simulink model "LeaderFollower"  (R2016a)
settings: Solver=VariableStepAuto  StartTime=0.0  StopTime=inf  RelTol=1e-3
settings Model: Creator=ece446  LastModifiedBy=ece446

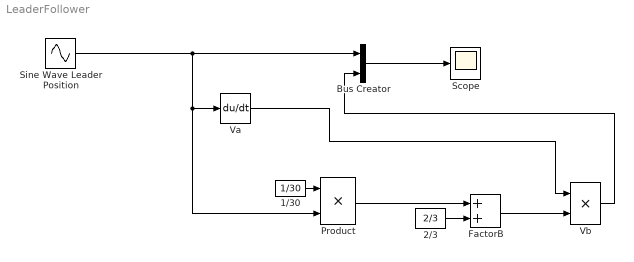
== system LeaderFollower ==
  1/30 : Constant  Value=1/30
  2/3 : Constant  Value=2/3
  Bus Creator : BusCreator  Inputs=2
  FactorB : Sum
  Product : Product
  "Scope " : Scope
  Sine Wave Leader Position : Sin  SampleTime=0
  Va : Derivative  CoefficientInTFapproximation=0
  Vb : Product
  wires:
  Sine Wave Leader Position/1 -> Bus Creator/1, Product/2, Va/1
  Va/1 -> Vb/1
  1/30/1 -> Product/1
  Product/1 -> FactorB/1
  2/3/1 -> FactorB/2
  FactorB/1 -> Vb/2
  Vb/1 -> Bus Creator/2
  Bus Creator/1 -> "Scope "/1
